simulink model "PDControllerThetap"  (R2017a)
settings: Solver=VariableStepAuto  StartTime=0.0  StopTime=10.0  RelTol=1e-3
settings Model: Creator=DF_Local  LastModifiedBy=DF_Local

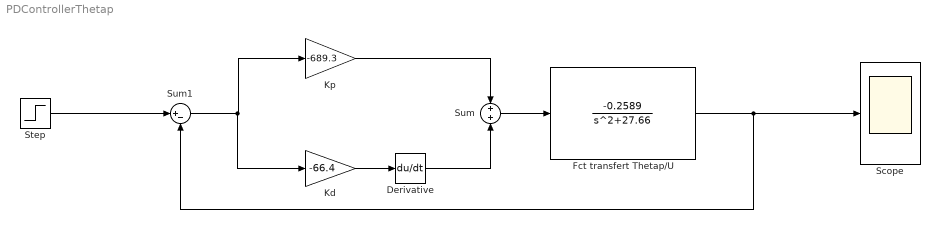
== system PDControllerThetap ==
  Derivative : Derivative
  Fct transfert Thetap/U : TransferFcn  Numerator=[-0.2589]  Denominator=[1 0 27.66]
  Kd : Gain  Gain=-66.4
  Kp : Gain  Gain=-689.3
  Scope : Scope
  Step : Step  Time=0  SampleTime=0
  Sum : Sum  Inputs=+|+
  Sum1 : Sum  Inputs=|+-
  wires:
  Sum1/1 -> Kd/1, Kp/1
  Kd/1 -> Derivative/1
  Kp/1 -> Sum/1
  Derivative/1 -> Sum/2
  Sum/1 -> Fct transfert Thetap/U/1
  Fct transfert Thetap/U/1 -> Scope/1, Sum1/2
  Step/1 -> Sum1/1
